simulink model "control_cdr_hybrid"  (Simulink 7.8)
settings: Solver=ode5  StartTime=0.0  StopTime=100  FixedStep=0.001  RelTol=1e-3
undefined symbols (not defined in the file): DamperOFF, DiscIntNeverNeededParam, Ki_L1, Ki_R1, Ki_R3, Kp_L1, Kp_R1, Kp_R2, Kp_R3, Matlab_version, Output_File, Output_file_n, Plant_inputs_num, Plant_outputs_num, polys, RecurDyn, RecurDyn_controltimestep, RecurDyn_model, RecurDyn_model_n, sigbuilder_block, SpringOFF, StaticTorque_RW1, StaticTorque_RW2, Ts, Tuning, Wheel_Vel
(part 2 of 2)

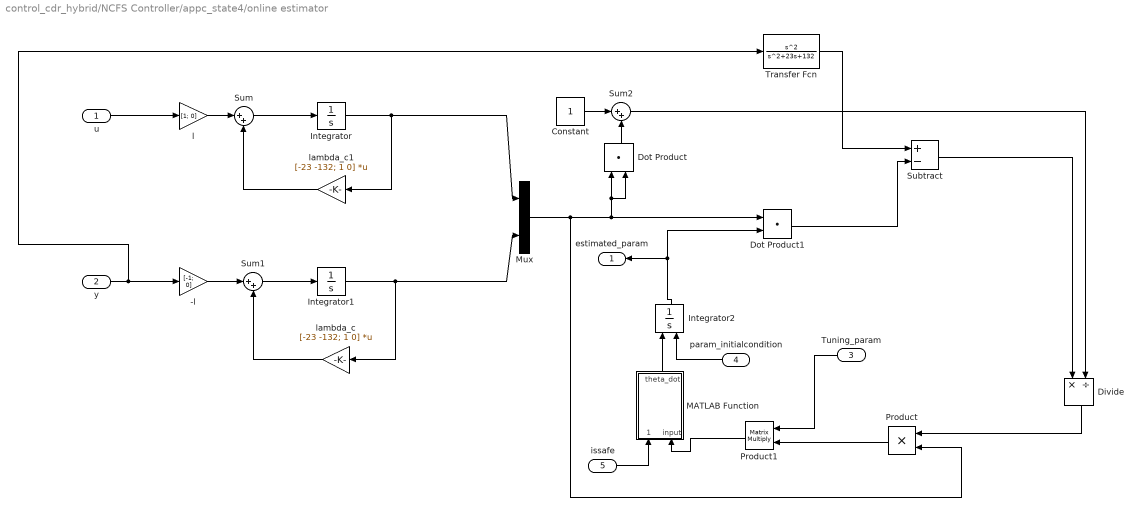
== system control_cdr_hybrid/NCFS Controller/appc_state4/online estimator ==
  u : Inport
  y : Inport  Port=2
  Tuning_param : Inport  Port=3
  param_initialcondition : Inport  Port=4
  issafe : Inport  Port=5
  -l : Gain  Gain=[-1; 0]
  Constant : Constant
  Divide : Product  Inputs=*/
  Dot Product : DotProduct  InputSameDT=on  OutDataTypeStr=Inherit: Inherit via internal rule
  Dot Product1 : DotProduct  InputSameDT=on  OutDataTypeStr=Inherit: Inherit via internal rule
  Integrator : Integrator
  Integrator1 : Integrator
  Integrator2 : Integrator  InitialConditionSource=external  InitialCondition=[1; 2; 4; 3]
  MATLAB Function : MATLAB Function  TreatAsAtomicUnit=on
  Mux : Mux  Inputs=2
  Product : Product  RndMeth=Zero
  Product1 : Product  Multiplication=Matrix(*)  RndMeth=Zero
  Subtract : Sum  Inputs=+-
  Sum : Sum  Inputs=|++
  Sum1 : Sum  Inputs=|++
  Sum2 : Sum  Inputs=|++
  Transfer Fcn : TransferFcn  Numerator=[1 0 0]  Denominator=[1 23 132]
  l : Gain  Gain=[1; 0]
  lambda_c : Gain  Gain=[-23 -132; 1 0]  Multiplication=Matrix(K*u)
  lambda_c1 : Gain  Gain=[-23 -132; 1 0]  Multiplication=Matrix(K*u)
  estimated_param : Outport
  wires:
  y/1 -> -l/1, Transfer Fcn/1
  u/1 -> l/1
  -l/1 -> Sum1/1
  l/1 -> Sum/1
  Sum/1 -> Integrator/1
  Integrator1/1 -> lambda_c/1, Mux/2
  Integrator/1 -> lambda_c1/1, Mux/1
  lambda_c1/1 -> Sum/2
  lambda_c/1 -> Sum1/2
  Mux/1 -> Dot Product/1, Dot Product/2, Dot Product1/1, Product/2
  Constant/1 -> Sum2/1
  Dot Product/1 -> Sum2/2
  Transfer Fcn/1 -> Subtract/1
  Dot Product1/1 -> Subtract/2
  Subtract/1 -> Divide/1
  Sum2/1 -> Divide/2
  Divide/1 -> Product/1
  Integrator2/1 -> Dot Product1/2, estimated_param/1
  Sum1/1 -> Integrator1/1
  Tuning_param/1 -> Product1/1
  Product/1 -> Product1/2
  param_initialcondition/1 -> Integrator2/2
  MATLAB Function/1(theta_dot) -> Integrator2/1
  issafe/1 -> MATLAB Function/1(issafe)
  Product1/1 -> MATLAB Function/2(input)

== system control_cdr_hybrid/Vehicle/RecurDyn Client Block/RecurDyn Plant ==
  " RecurDyn_inputs" : Inport
  S-Function : S-Function  FunctionName=recurdyn_client_7_13  Parameters=RecurDyn_controltimestep_,RecurDyn_model_name,RecurDyn_,RecurDyn_static_,RecurDyn_step_,RecurDyn_show_,RecurDyn_ani_,Matlab_version_,RecurDyn_model_n,Plant_inputs_num,Plant_outputs_num,Waitingtime,Create_Output_Folder_,Output_File_Name_,Output_file_n  EnableBusSupport=off
  RecurDyn_outputs : Outport  InitialOutput=0
  wires:
  S-Function/1 -> RecurDyn_outputs/1
  " RecurDyn_inputs"/1 -> S-Function/1

== system control_cdr_hybrid/Vehicle Velocity Controller (Driver Model)/L1_controller/Subsystem ==
  In1 : Inport
  Discrete-Time Integrator : DiscreteIntegrator  SampleTime=Ts  LimitOutput=on  UpperSaturationLimit=100  LowerSaturationLimit=-100  ICPrevOutput=DiscIntNeverNeededParam  ICPrevScaledInput=DiscIntNeverNeededParam
  Kp4 : Gain  Gain=Kp_L1  SampleTime=Ts  SaturateOnIntegerOverflow=on  OutDataTypeStr=Inherit: Same as input  ParamDataTypeStr=Inherit: Same as input
  Kp5 : Gain  Gain=Ki_L1  SampleTime=Ts  SaturateOnIntegerOverflow=on  OutDataTypeStr=Inherit: Same as input  ParamDataTypeStr=Inherit: Same as input
  Sum6 : Sum  SampleTime=Ts  SaturateOnIntegerOverflow=on  InputSameDT=on  OutDataTypeStr=Inherit: Same as first input
  Zero-Order Hold : ZeroOrderHold  SampleTime=Ts
  Out1 : Outport
  wires:
  Sum6/1 -> Out1/1
  Zero-Order Hold/1 -> Sum6/1
  Discrete-Time Integrator/1 -> Sum6/2
  Kp4/1 -> Zero-Order Hold/1
  Kp5/1 -> Discrete-Time Integrator/1
  In1/1 -> Kp4/1, Kp5/1

== system control_cdr_hybrid/Vehicle Velocity Controller (Driver Model)/R1_controller/Subsystem ==
  In1 : Inport
  Discrete-Time Integrator : DiscreteIntegrator  SampleTime=Ts  LimitOutput=on  UpperSaturationLimit=100  LowerSaturationLimit=-100  ICPrevOutput=DiscIntNeverNeededParam  ICPrevScaledInput=DiscIntNeverNeededParam
  Kp4 : Gain  Gain=Kp_R1  SampleTime=Ts  SaturateOnIntegerOverflow=on  OutDataTypeStr=Inherit: Same as input  ParamDataTypeStr=Inherit: Same as input
  Kp5 : Gain  Gain=Ki_R1  SampleTime=Ts  SaturateOnIntegerOverflow=on  OutDataTypeStr=Inherit: Same as input  ParamDataTypeStr=Inherit: Same as input
  Sum6 : Sum  SampleTime=Ts  SaturateOnIntegerOverflow=on  InputSameDT=on  OutDataTypeStr=Inherit: Same as first input
  Zero-Order Hold : ZeroOrderHold  SampleTime=Ts
  Out1 : Outport
  wires:
  Sum6/1 -> Out1/1
  Zero-Order Hold/1 -> Sum6/1
  Discrete-Time Integrator/1 -> Sum6/2
  Kp4/1 -> Zero-Order Hold/1
  Kp5/1 -> Discrete-Time Integrator/1
  In1/1 -> Kp4/1, Kp5/1

== system control_cdr_hybrid/Vehicle Velocity Controller (Driver Model)/R2_controller/Subsystem ==
  In1 : Inport
  Discrete-Time Integrator : DiscreteIntegrator  SampleTime=Ts  LimitOutput=on  UpperSaturationLimit=100  LowerSaturationLimit=-100  ICPrevOutput=DiscIntNeverNeededParam  ICPrevScaledInput=DiscIntNeverNeededParam
  Kp4 : Gain  Gain=Kp_R2  SampleTime=Ts  SaturateOnIntegerOverflow=on  OutDataTypeStr=Inherit: Same as input  ParamDataTypeStr=Inherit: Same as input
  Kp5 : Gain  Gain=Ki_R1  SampleTime=Ts  SaturateOnIntegerOverflow=on  OutDataTypeStr=Inherit: Same as input  ParamDataTypeStr=Inherit: Same as input
  Sum6 : Sum  SampleTime=Ts  SaturateOnIntegerOverflow=on  InputSameDT=on  OutDataTypeStr=Inherit: Same as first input
  Zero-Order Hold : ZeroOrderHold  SampleTime=Ts
  Out1 : Outport
  wires:
  Sum6/1 -> Out1/1
  Zero-Order Hold/1 -> Sum6/1
  Discrete-Time Integrator/1 -> Sum6/2
  Kp4/1 -> Zero-Order Hold/1
  Kp5/1 -> Discrete-Time Integrator/1
  In1/1 -> Kp4/1, Kp5/1

== system control_cdr_hybrid/Vehicle Velocity Controller (Driver Model)/R3_controller/Subsystem ==
  In1 : Inport
  Discrete-Time Integrator : DiscreteIntegrator  SampleTime=Ts  LimitOutput=on  UpperSaturationLimit=100  LowerSaturationLimit=-100  ICPrevOutput=DiscIntNeverNeededParam  ICPrevScaledInput=DiscIntNeverNeededParam
  Kp4 : Gain  Gain=Kp_R3  SampleTime=Ts  SaturateOnIntegerOverflow=on  OutDataTypeStr=Inherit: Same as input  ParamDataTypeStr=Inherit: Same as input
  Kp5 : Gain  Gain=Ki_R3  SampleTime=Ts  SaturateOnIntegerOverflow=on  OutDataTypeStr=Inherit: Same as input  ParamDataTypeStr=Inherit: Same as input
  Sum6 : Sum  SampleTime=Ts  SaturateOnIntegerOverflow=on  InputSameDT=on  OutDataTypeStr=Inherit: Same as first input
  Zero-Order Hold : ZeroOrderHold  SampleTime=Ts
  Out1 : Outport
  wires:
  Sum6/1 -> Out1/1
  Zero-Order Hold/1 -> Sum6/1
  Discrete-Time Integrator/1 -> Sum6/2
  Kp4/1 -> Zero-Order Hold/1
  Kp5/1 -> Discrete-Time Integrator/1
  In1/1 -> Kp4/1, Kp5/1

== matlab function NCFS Controller/appc_state3/adaptive_interface_con/A_hat ==
  data: e_hat input double; out output double; theta_1 input double; A_hat output double
function [out,A_hat] = A_hat(e_hat,theta_1)
%#codegen

% theta_1=theta_a

A_hat=[-theta_1 [1 0; 0 1; 0 0]];
out=A_hat*e_hat;

== matlab function NCFS Controller/MATLAB Function ==
  data: init_time input double; time output double; issafe output double
function [time,issafe] = fcn(init_time)
%#codegen

if (init_time > 0)
    time=init_time-1;
    issafe=1;
else
    time=0;
    issafe=0;
end

== matlab function NCFS Controller/appc_state3/adaptive_interface_con/change ==
  data: theta_1 output double; theta_a input double
function theta_1  = change(theta_a)
%#codegen

theta_1=[theta_a; 0];

== matlab function NCFS Controller/appc_state3/adaptive_interface_con/change2 ==
  data: theta_2 output double; theta_b input double
function theta_2  = change(theta_b)
%#codegen

theta_2 = [theta_b; 0]+2*[0; theta_b];

== matlab function NCFS Controller/appc_state3/adaptive_interface_con/feedback ==
  data: e_hat input double; A_hat input double; out output double; B_hat input double; Poly input double
function out = control(e_hat,A_hat,B_hat,Poly)
%#codegen

% theta_1=theta_a
K_c=[0 0 1]*[B_hat A_hat*B_hat A_hat^2*B_hat]^(-1)*(A_hat^3+Poly(2)*A_hat^2+Poly(3)*A_hat+Poly(4)*eye(3));
out=-K_c*e_hat;

== matlab function NCFS Controller/appc_state3/adaptive_interface_con/observ ==
  data: theta_1 input double; input input double; out output double; K_o output double
function [out, K_o] =observ(theta_1,input)
%#codegen


K_o=[25;191;455]-theta_1;
out=K_o*input;

== matlab function NCFS Controller/appc_state3/adaptive_interface_con/statechoose ==
  data: x1 input double; x2 input double; state output double; x3 input double; ym_des input double; ym_des_before input double; change output double; ym_des_mem output double
function [state,change,ym_des_mem] = statechoose(x1,x2,x3,ym_des,ym_des_before)
%#codegen

if (not(ym_des_before == ym_des)) % ym_des changed
    change = 1;
    if(0.5<= ym_des <= 1)
        state=(ym_des-0.5)*x1/0.5+(1-ym_des)*x2/0.5;
    elseif(0 <= ym_des <= 0.5)
        state=(ym_des)*x2/0.5+(0.5-ym_des)*x3/0.5;
    else
        state=[0;0;0];
        
    end
else
    change = 0;
    state = [0;0;0]; % null, has no meaning
end

ym_des_mem=ym_des;

== matlab function NCFS Controller/appc_state3/adaptive_interface_con/transpose1 ==
  data: u input double; theta_b output double; theta_a output double
function [theta_b,theta_a] = demux(u)
%#codegen

theta_b = u(1:2);
theta_a = u(3:4);

== matlab function NCFS Controller/appc_state4/adaptive_interface_con/A_hat ==
  data: e_hat input double; out output double; theta_1 input double; A_hat output double
function [out,A_hat] = A_hat(e_hat,theta_1)
%#codegen

% theta_1=theta_a

A_hat=[-theta_1 [1 0; 0 1; 0 0]];
out=A_hat*e_hat;

== matlab function NCFS Controller/appc_state4/adaptive_interface_con/change ==
  data: theta_1 output double; theta_a input double
function theta_1  = change(theta_a)
%#codegen

theta_1=[theta_a; 0];

== matlab function NCFS Controller/appc_state4/adaptive_interface_con/change2 ==
  data: theta_2 output double; theta_b input double
function theta_2  = change(theta_b)
%#codegen

theta_2 = [theta_b; 0]+2*[0; theta_b];

== matlab function NCFS Controller/appc_state4/adaptive_interface_con/feedback ==
  data: e_hat input double; A_hat input double; out output double; B_hat input double; Poly input double
function out = control(e_hat,A_hat,B_hat,Poly)
%#codegen

% theta_1=theta_a
K_c=[0 0 1]*[B_hat A_hat*B_hat A_hat^2*B_hat]^(-1)*(A_hat^3+Poly(2)*A_hat^2+Poly(3)*A_hat+Poly(4)*eye(3));
out=-K_c*e_hat;

== matlab function NCFS Controller/appc_state4/adaptive_interface_con/observ ==
  data: theta_1 input double; input input double; out output double; K_o output double
function [out, K_o] =observ(theta_1,input)
%#codegen


K_o=[25;191;455]-theta_1;
out=K_o*input;

== matlab function NCFS Controller/appc_state4/adaptive_interface_con/statechoose ==
  data: x1 input double; x2 input double; state output double; x3 input double; ym_des input double; ym_des_before input double; change output double; ym_des_mem output double
function [state,change,ym_des_mem] = statechoose(x1,x2,x3,ym_des,ym_des_before)
%#codegen

if (not(ym_des_before == ym_des)) % ym_des changed
    change = 1;
    if(0.5<= ym_des <= 1)
        state=(ym_des-0.5)*x1/0.5+(1-ym_des)*x2/0.5;
    elseif(0 <= ym_des <= 0.5)
        state=(ym_des)*x2/0.5+(0.5-ym_des)*x3/0.5;
    else
        state=[0;0;0];
        
    end
else
    change = 0;
    state = [0;0;0]; % null, has no meaning
end

ym_des_mem=ym_des;

== matlab function NCFS Controller/appc_state4/adaptive_interface_con/transpose1 ==
  data: u input double; theta_b output double; theta_a output double
function [theta_b,theta_a] = demux(u)
%#codegen

theta_b = u(1:2);
theta_a = u(3:4);

== matlab function NCFS Controller/MATLAB Function1 ==
  data: pitch_acc input double; d_ym1 output double; d_ym2 output double; hull_acc input double
function [d_ym1,d_ym2] = judge(pitch_acc,hull_acc)
%#codegen

if (abs(hull_acc)>1500)
    t_hull_acc=1500*sign(hull_acc);
else
    t_hull_acc=hull_acc;
end
del_theta=(tan(-t_hull_acc/1500*0.8)/tan(0.8)*0.4);

if (del_theta<-0.2)
    d_ym1_1=-0.2;
elseif(del_theta>0.4)
    d_ym1_1=0.4;
else
    d_ym1_1=del_theta;
end

if (del_theta<-0.3189)
    d_ym2_1=-0.3189;
elseif(del_theta>0.3)
    d_ym2_1=0.3;
else
    d_ym2_1=del_theta;
end

if (abs(pitch_acc)>2)
    t_pitch_acc=2*sign(pitch_acc);
else
    t_pitch_acc=pitch_acc;
end

del_theta_2=(tan(-t_pitch_acc/2*0.8)/tan(0.8)*0.4);

if (del_theta_2<-0.2)
    d_ym1_2=-0.2;
elseif(del_theta_2>0.4)
    d_ym1_2=0.4;
else
    d_ym1_2=del_theta_2;
end

if (del_theta_2<-0.3189)
    d_ym2_2=-0.3189;
elseif(del_theta_2>0.3)
    d_ym2_2=0.3;
else
    d_ym2_2=del_theta_2;
end

d_ym1=d_ym1_1+d_ym1_2;
d_ym2=d_ym2_1+d_ym2_2;

% if (d_ym1<-0.2)
%     d_ym1=-0.2;
% elseif(d_ym1>0.4)
%     d_ym1=0.4;
% end
% 
% if (d_ym2<-0.3189)
%     d_ym2=-0.3189;
% elseif(d_ym2>0.3)
%     d_ym2=0.3;
% end

d_ym2=-d_ym2;
d_ym1=d_ym1*8;
d_ym2=d_ym2*8;

== matlab function NCFS Controller/appc_state2/online estimator/MATLAB Function ==
  data: issafe input double; theta_dot output double; input input double
function theta_dot = switch_input(issafe,input)
%#codegen

issafe=~issafe;
theta_dot=issafe*input;

== matlab function NCFS Controller/appc_state1/adaptive_interface_con/A_hat ==
  data: e_hat input double; out output double; theta_1 input double; A_hat output double
function [out,A_hat] = A_hat(e_hat,theta_1)
%#codegen

% theta_1=theta_a

A_hat=[-theta_1 [1 0; 0 1; 0 0]];
out=A_hat*e_hat;

== matlab function NCFS Controller/appc_state1/adaptive_interface_con/change ==
  data: theta_1 output double; theta_a input double
function theta_1  = change(theta_a)
%#codegen

theta_1=[theta_a; 0];

== matlab function NCFS Controller/appc_state1/adaptive_interface_con/change2 ==
  data: theta_2 output double; theta_b input double
function theta_2  = change(theta_b)
%#codegen

theta_2 = [theta_b; 0]+2*[0; theta_b];

== matlab function NCFS Controller/appc_state1/adaptive_interface_con/feedback ==
  data: e_hat input double; A_hat input double; out output double; B_hat input double; Poly input double
function out = control(e_hat,A_hat,B_hat,Poly)
%#codegen

% theta_1=theta_a
K_c=[0 0 1]*[B_hat A_hat*B_hat A_hat^2*B_hat]^(-1)*(A_hat^3+Poly(2)*A_hat^2+Poly(3)*A_hat+Poly(4)*eye(3));
out=-K_c*e_hat;

== matlab function NCFS Controller/appc_state1/adaptive_interface_con/observ ==
  data: theta_1 input double; input input double; out output double; K_o output double
function [out, K_o] =observ(theta_1,input)
%#codegen


K_o=[25;191;455]-theta_1;
out=K_o*input;

== matlab function NCFS Controller/appc_state1/adaptive_interface_con/statechoose ==
  data: x1 input double; x2 input double; state output double; x3 input double; ym_des input double; ym_des_before input double; change output double; ym_des_mem output double
function [state,change,ym_des_mem] = statechoose(x1,x2,x3,ym_des,ym_des_before)
%#codegen

if (not(ym_des_before == ym_des)) % ym_des changed
    change = 1;
    if(0.5<= ym_des <= 1)
        state=(ym_des-0.5)*x1/0.5+(1-ym_des)*x2/0.5;
    elseif(0 <= ym_des <= 0.5)
        state=(ym_des)*x2/0.5+(0.5-ym_des)*x3/0.5;
    else
        state=[0;0;0];
        
    end
else
    change = 0;
    state = [0;0;0]; % null, has no meaning
end

ym_des_mem=ym_des;

== matlab function NCFS Controller/appc_state1/adaptive_interface_con/transpose1 ==
  data: u input double; theta_b output double; theta_a output double
function [theta_b,theta_a] = demux(u)
%#codegen

theta_b = u(1:2);
theta_a = u(3:4);

== matlab function NCFS Controller/appc_state2/adaptive_interface_con1/A_hat ==
  data: e_hat input double; out output double; theta_1 input double; A_hat output double
function [out,A_hat] = A_hat(e_hat,theta_1)
%#codegen

% theta_1=theta_a

A_hat=[-theta_1 [1 0; 0 1; 0 0]];
out=A_hat*e_hat;

== matlab function NCFS Controller/appc_state1/online estimator/MATLAB Function ==
  data: issafe input double; theta_dot output double; input input double
function theta_dot = switch_input(issafe,input)
%#codegen

issafe=~issafe;
theta_dot=issafe*input;

== matlab function NCFS Controller/appc_state3/online estimator/MATLAB Function ==
  data: issafe input double; theta_dot output double; input input double
function theta_dot = switch_input(issafe,input)
%#codegen

issafe=~issafe;
theta_dot=issafe*input;

== matlab function NCFS Controller/appc_state2/adaptive_interface_con1/change ==
  data: theta_1 output double; theta_a input double
function theta_1  = change(theta_a)
%#codegen

theta_1=[theta_a; 0];

== matlab function NCFS Controller/appc_state2/adaptive_interface_con1/change2 ==
  data: theta_2 output double; theta_b input double
function theta_2  = change(theta_b)
%#codegen

theta_2 = [theta_b; 0]+2*[0; theta_b];

== matlab function NCFS Controller/appc_state2/adaptive_interface_con1/feedback ==
  data: e_hat input double; A_hat input double; out output double; B_hat input double; Poly input double
function out = control(e_hat,A_hat,B_hat,Poly)
%#codegen

% theta_1=theta_a
K_c=[0 0 1]*[B_hat A_hat*B_hat A_hat^2*B_hat]^(-1)*(A_hat^3+Poly(2)*A_hat^2+Poly(3)*A_hat+Poly(4)*eye(3));
out=-K_c*e_hat;

== matlab function NCFS Controller/appc_state2/adaptive_interface_con1/observ ==
  data: theta_1 input double; input input double; out output double; K_o output double
function [out, K_o] =observ(theta_1,input)
%#codegen


K_o=[25;191;455]-theta_1;
out=K_o*input;

== matlab function NCFS Controller/appc_state2/adaptive_interface_con1/statechoose ==
  data: x1 input double; x2 input double; state output double; x3 input double; ym_des input double; ym_des_before input double; change output double; ym_des_mem output double
function [state,change,ym_des_mem] = statechoose(x1,x2,x3,ym_des,ym_des_before)
%#codegen

if (not(ym_des_before == ym_des)) % ym_des changed
    change = 1;
    if(0.5<= ym_des <= 1)
        state=(ym_des-0.5)*x1/0.5+(1-ym_des)*x2/0.5;
    elseif(0 <= ym_des <= 0.5)
        state=(ym_des)*x2/0.5+(0.5-ym_des)*x3/0.5;
    else
        state=[0;0;0];
        
    end
else
    change = 0;
    state = [0;0;0]; % null, has no meaning
end

ym_des_mem=ym_des;

== matlab function NCFS Controller/appc_state2/adaptive_interface_con1/transpose1 ==
  data: u input double; theta_b output double; theta_a output double
function [theta_b,theta_a] = demux(u)
%#codegen

theta_b = u(1:2);
theta_a = u(3:4);

== matlab function NCFS Controller/appc_state4/online estimator/MATLAB Function ==
  data: issafe input double; theta_dot output double; input input double
function theta_dot = switch_input(issafe,input)
%#codegen

issafe=~issafe;
theta_dot=issafe*input;
